simulink model "gm_sampleModel1426_2_sub"  (R2023a)
settings: Solver=VariableStepAuto  StartTime=0.0  StopTime=10.0  RelTol=1e-3
libraries: simulink x2, hdlsllib x1
settings Model: Creator=user1  LastModifiedBy=user1
settings OptimizationCC: BlockReduction=off  ConditionallyExecuteInputs=off
settings DebuggingCC: InheritedTsInSrcMsg=none

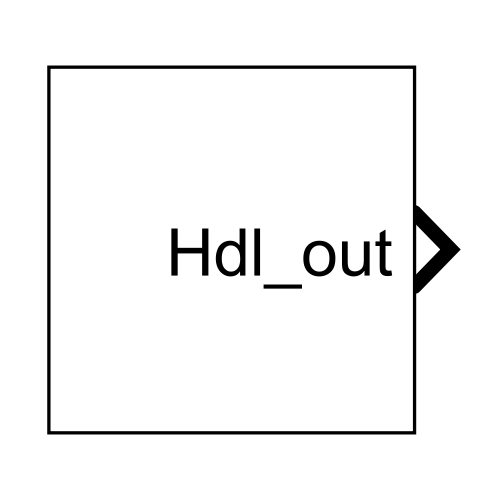
[thumbnail: Simulink's stored preview of the top-level diagram]
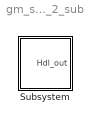
== system gm_sampleModel1426_2_sub ==
  Subsystem : Subsystem

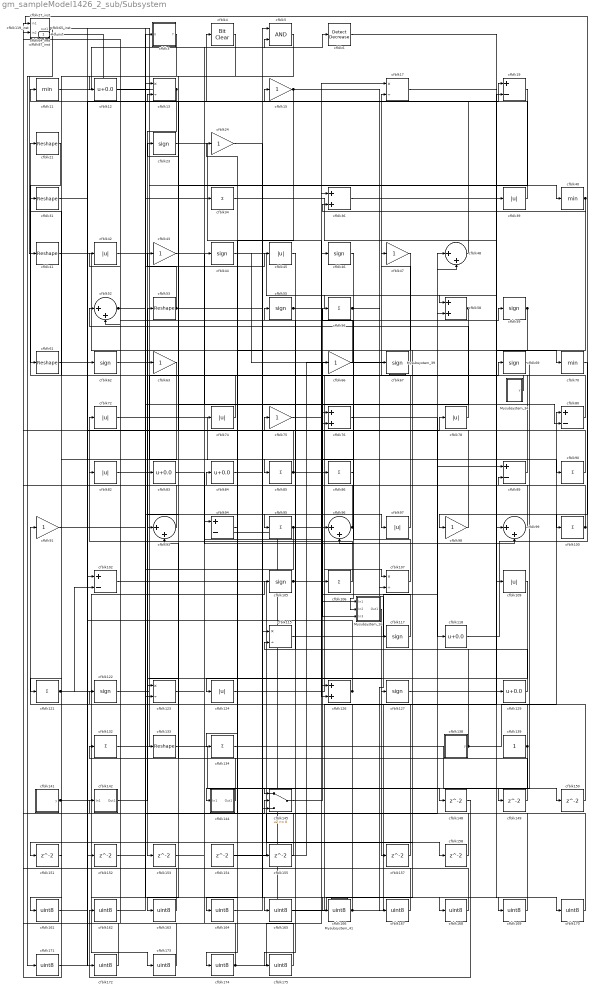
== system gm_sampleModel1426_2_sub/Subsystem ==
  Mysubsystem_16 : Subsystem
  Mysubsystem_34 : Subsystem
  Mysubsystem_39 : Subsystem
  Mysubsystem_41 : Subsystem
  cfblk{34,56,85..86,90,95,100,106,121,132,134} (11 alike) : Sum  Inputs=+  OutDataTypeStr=uint8
  cfblk{19,80,89,94,102} (5 alike) : Sum  Inputs=+-  OutDataTypeStr=uint8
  cfblk{23,44,46,55,59,62,67,69,105,117,122,127} (12 alike) : Signum
  cfblk{13,17,107,115,123} (5 alike) : Product  Inputs=*/  OutDataTypeStr=uint8  RndMeth=Zero  SaturateOnIntegerOverflow=on
  cfblk{39,42,45,72,74,78,82,97,109,124} (10 alike) : Abs  OutDataTypeStr=uint8  SaturateOnIntegerOverflow=off
  cfblk11 : MinMax  OutDataTypeStr=uint8
  cfblk111_inst : Subsystem
  cfblk{12,83..84,118,129} (5 alike) : Bias  Bias=0.0  SaturateOnIntegerOverflow=off
  cfblk119_inst : Subsystem
  cfblk{36,58,76,126} (4 alike) : Sum  OutDataTypeStr=uint8
  cfblk{21,31,41,53,61,133} (6 alike) : Reshape
  cfblk138 : Subsystem  mask(Counter Limited){uplimit=double(7), tsamp=double(-1)}
      mask prompts: uplimit "Simulink:masks:UpperLimit_MP"; tsamp "Simulink:masks:SampleTime_MP"
      mask help: Simulink:masks:CounterLimited_MD
      mask init:
      | nbits = double(8);
      | tsamp = double(-1);
      | uplimit = double(7);
  cfblk139 : Constant  OutDataTypeStr=uint8  SampleTime=-1
  cfblk141 : Subsystem  mask(Counter Free-Running){NumBits=double(16), tsamp=double(-1)}
      mask prompts: NumBits "Simulink:masks:NumberOfBits_MP"; tsamp "Simulink:masks:SampleTime_MP"
      mask help: Simulink:masks:CounterFreeRunning_MD
  cfblk142 : Subsystem
  cfblk144 : Subsystem
  cfblk145 : Switch  OutDataTypeStr=uint8  SaturateOnIntegerOverflow=off  InputSameDT=off
  cfblk{148..155,157..158} (10 alike) : Delay  SampleTime=1
  cfblk{15,24,43,47,63,66,75,91,98} (9 alike) : Gain  OutDataTypeStr=uint8
  cfblk{161..175} (15 alike) : DataTypeConversion  OutDataTypeStr=uint8  SaturateOnIntegerOverflow=off  RndMeth=Floor
  cfblk27_inst : Subsystem
  cfblk3 : Subsystem  mask(Detect Rise Positive){vinit=double(0), InputProcessing=Elements as channels (sample based), OutDataTypeStr=uint8}
      mask prompts: vinit "Simulink:masks:InitialCondition_MP"; InputProcessing "Simulink:masks:InputProcessing_MP"; OutDataTypeStr "Simulink:masks:OutputDataType_MP"
      mask help: Simulink:masks:DetectRisePositive_MD
      mask init:
      | InputProcessing = 'Elements as channels (sample based)';
      | OutDataTypeStr = 'uint8';
      | vinit = double(0);
      mask TypeOptions InputProcessing: Simulink:masks:ColumnsAsChannelsFrameBased | Simulink:masks:ElementsAsChannelsSampleBased
      mask TypeOptions OutDataTypeStr: Simulink:masks:uint8 | Simulink:masks:boolean
      mask Display: fprintf('U > 0\n&  NOT\nU/z > 0')
  cfblk4 : simulink/Logic and Bit Operations/Bit Clear  iBit=0
      settings: LibrarySourceBlock=|
      | hdlsllib/Logic and Bit
      | Operations/Bit Clear
  cfblk40 : MinMax  OutDataTypeStr=uint8
  cfblk{48,52,93,96,99} (5 alike) : Sum  Inputs=|++  OutDataTypeStr=uint8
  cfblk5 : Logic  AllPortsSameDT=off  OutDataTypeStr=boolean
  cfblk6 : simulink/Logic and Bit Operations/Detect Decrease  vinit=0.0  OutDataTypeStr=uint8
      settings: LibrarySourceBlock=|
      | hdlsllib/Logic and Bit
      | Operations/Detect
      | Decrease
  cfblk64_inst : Subsystem
  cfblk65_inst : Subsystem
  cfblk70 : MinMax  OutDataTypeStr=uint8
  cfblk87_inst : Subsystem
  Hdl_out : Outport  OutDataTypeStr=uint8  SampleTime=1
  wires:
  Mysubsystem_16/1(Out1) -> cfblk151/1
  Mysubsystem_34/1(y) -> cfblk21/1
  Mysubsystem_39/1(Out1) -> cfblk154/1
  Mysubsystem_41/1(Out1) -> cfblk94/2
  cfblk100/1 -> cfblk89/2, cfblk98/1
  cfblk102/1 -> cfblk158/1
  cfblk105/1 -> cfblk107/1, Mysubsystem_16/3(In3)
  cfblk106/1 -> cfblk72/1
  cfblk107/1 -> cfblk75/1
  cfblk109/1 -> cfblk124/1
  cfblk11/1 -> cfblk5/2
  cfblk111_inst/1(out1) -> cfblk171/1
  cfblk115/1 -> cfblk48/1
  cfblk117/1 -> cfblk66/1
  cfblk118/1 -> cfblk87_inst/1(in1)
  cfblk119_inst/1(out1) -> cfblk85/1
  cfblk12/1 -> cfblk40/1
  cfblk121/1 -> cfblk105/1, cfblk102/2
  cfblk122/1 -> cfblk127/1
  cfblk123/1 -> cfblk6/1
  cfblk124/1 -> cfblk17/2
  cfblk126/1 -> cfblk46/1, cfblk102/1
  cfblk127/1 -> cfblk39/1
  cfblk129/1 -> cfblk115/2
  cfblk13/1 -> cfblk153/1, Hdl_out/1
  cfblk132/1 -> cfblk67/1
  cfblk133/1 -> cfblk148/1
  cfblk134/1 -> cfblk150/1
  cfblk138/1(y) -> cfblk80/1, cfblk55/1
  cfblk139/1 -> cfblk52/2, cfblk144/1(In1)
  cfblk141/1(y) -> cfblk44/1, cfblk173/1, cfblk168/1, cfblk165/1
  cfblk142/1(Out1) -> cfblk53/1
  cfblk144/1(Out1) -> cfblk132/1
  cfblk145/1 -> cfblk106/1
  cfblk148/1 -> cfblk162/1
  cfblk149/1 -> cfblk93/2
  cfblk15/1 -> cfblk164/1, cfblk107/2
  cfblk150/1 -> cfblk126/1
  cfblk151/1 -> cfblk119_inst/2(in2)
  cfblk152/1 -> cfblk145/2
  cfblk153/1 -> cfblk96/1
  cfblk154/1 -> cfblk48/2
  cfblk155/1 -> cfblk27_inst/1(in1)
  cfblk157/1 -> cfblk115/1
  cfblk158/1 -> cfblk5/1
  cfblk161/1 -> cfblk78/1
  cfblk162/1 -> cfblk3/1(U)
  cfblk163/1 -> cfblk87_inst/2(in2)
  cfblk164/1 -> cfblk19/1
  cfblk165/1 -> cfblk19/2
  cfblk166/1 -> cfblk58/2, cfblk91/1
  cfblk167/1 -> cfblk64_inst/1(in1)
  cfblk168/1 -> cfblk64_inst/2(in2)
  cfblk169/1 -> cfblk142/1(In1)
  cfblk17/1 -> cfblk170/1
  cfblk170/1 -> cfblk84/1
  cfblk171/1 -> cfblk62/1
  cfblk172/1 -> cfblk111_inst/1(in1)
  cfblk173/1 -> cfblk111_inst/2(in2)
  cfblk174/1 -> cfblk76/2, cfblk122/1
  cfblk175/1 -> cfblk94/1
  cfblk19/1 -> cfblk163/1
  cfblk21/1 -> cfblk61/1
  cfblk23/1 -> cfblk126/2
  cfblk24/1 -> cfblk155/1
  cfblk27_inst/1(out1) -> cfblk65_inst/2(in2), cfblk41/1
  cfblk3/1(Y) -> cfblk161/1
  cfblk31/1 -> cfblk172/1
  cfblk34/1 -> cfblk129/1
  cfblk36/1 -> cfblk70/1
  cfblk39/1 -> cfblk4/1
  cfblk4/1 -> cfblk12/1
  cfblk40/1 -> cfblk36/2, Mysubsystem_41/1(In1)
  cfblk41/1 -> cfblk145/3
  cfblk42/1 -> Mysubsystem_39/1(In1)
  cfblk43/1 -> cfblk76/1
  cfblk44/1 -> cfblk109/1
  cfblk45/1 -> cfblk175/1
  cfblk46/1 -> cfblk86/1
  cfblk47/1 -> cfblk145/1
  cfblk48/1 -> cfblk11/1
  cfblk5/1 -> cfblk93/1
  cfblk52/1 -> cfblk83/1, cfblk80/2, cfblk34/1
  cfblk53/1 -> cfblk97/1, cfblk43/1
  cfblk55/1 -> cfblk58/1, Mysubsystem_16/1(In1)
  cfblk56/1 -> cfblk167/1, cfblk117/1
  cfblk58/1 -> cfblk157/1, cfblk123/1
  cfblk59/1 -> Mysubsystem_16/2(In2), cfblk134/1
  cfblk6/1 -> cfblk99/1
  cfblk61/1 -> cfblk15/1
  cfblk62/1 -> cfblk90/1
  cfblk63/1 -> cfblk121/1
  cfblk64_inst/1(out1) -> cfblk166/1
  cfblk65_inst/1(out1) -> cfblk152/1, cfblk95/1
  cfblk66/1 -> cfblk119_inst/1(in1)
  cfblk67/1 -> cfblk47/1
  cfblk69/1 -> cfblk149/1
  cfblk70/1 -> cfblk100/1
  cfblk72/1 -> cfblk118/1
  cfblk74/1 -> cfblk63/1
  cfblk75/1 -> cfblk17/1
  cfblk76/1 -> cfblk89/1
  cfblk78/1 -> cfblk52/1
  cfblk80/1 -> cfblk13/2
  cfblk82/1 -> cfblk133/1
  cfblk83/1 -> cfblk99/2
  cfblk84/1 -> cfblk169/1
  cfblk85/1 -> cfblk69/1, cfblk65_inst/1(in1), cfblk59/1
  cfblk86/1 -> cfblk96/2
  cfblk87_inst/1(out1) -> cfblk74/1
  cfblk89/1 -> cfblk42/1
  cfblk90/1 -> cfblk23/1
  cfblk91/1 -> cfblk45/1
  cfblk93/1 -> cfblk27_inst/2(in2)
  cfblk94/1 -> cfblk174/1
  cfblk95/1 -> cfblk36/1, cfblk123/2
  cfblk96/1 -> cfblk82/1, cfblk56/1
  cfblk97/1 -> cfblk31/1
  cfblk98/1 -> cfblk13/1
  cfblk99/1 -> cfblk24/1

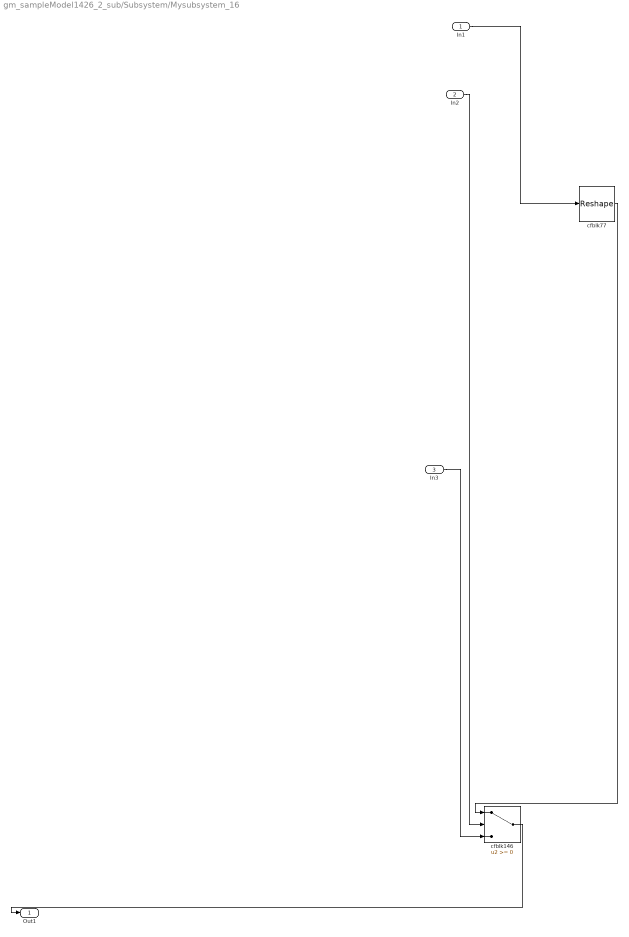
== system gm_sampleModel1426_2_sub/Subsystem/Mysubsystem_16 ==
  In1 : Inport  OutDataTypeStr=uint8  PortDimensions=1  SampleTime=1
  In2 : Inport  Port=2  OutDataTypeStr=uint8  PortDimensions=1  SampleTime=1
  In3 : Inport  Port=3  OutDataTypeStr=uint8  PortDimensions=1  SampleTime=1
  cfblk146 : Switch  SaturateOnIntegerOverflow=off  InputSameDT=off
  cfblk77 : Reshape
  Out1 : Outport  SampleTime=1
  wires:
  In1/1 -> cfblk77/1
  In2/1 -> cfblk146/2
  In3/1 -> cfblk146/3
  cfblk146/1 -> Out1/1
  cfblk77/1 -> cfblk146/1

== system gm_sampleModel1426_2_sub/Subsystem/Mysubsystem_34 ==
  cfblk140 : Subsystem  mask(Counter Free-Running){NumBits=double(16), tsamp=double(-1)}
      mask prompts: NumBits "Simulink:masks:NumberOfBits_MP"; tsamp "Simulink:masks:SampleTime_MP"
      mask help: Simulink:masks:CounterFreeRunning_MD
  cfblk8 : hdlsllib/Logic and Bit Operations/Interval Test  IntervalClosedRight=on  uplimit=0.5  IntervalClosedLeft=on  lowlimit=-0.5  OutDataTypeStr=boolean
  y : Outport  SampleTime=1
  wires:
  cfblk140/1(y) -> cfblk8/1
  cfblk8/1 -> y/1

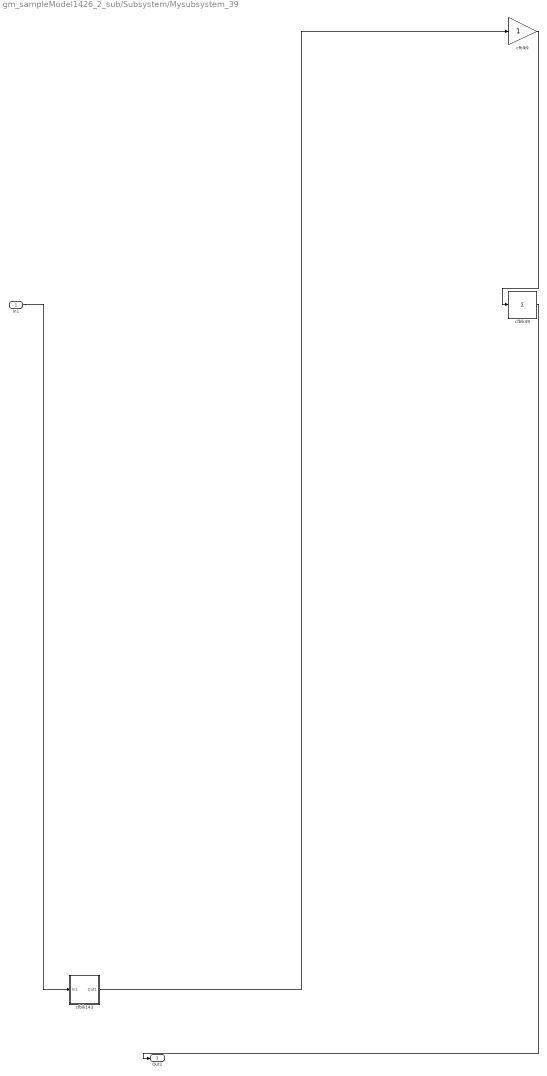
== system gm_sampleModel1426_2_sub/Subsystem/Mysubsystem_39 ==
  In1 : Inport  OutDataTypeStr=uint8  PortDimensions=1  SampleTime=1
  cfblk143 : Subsystem
  cfblk49 : Sum  Inputs=+
  cfblk9 : Gain
  Out1 : Outport  SampleTime=1
  wires:
  In1/1 -> cfblk143/1(In1)
  cfblk143/1(Out1) -> cfblk9/1
  cfblk49/1 -> Out1/1
  cfblk9/1 -> cfblk49/1

== system gm_sampleModel1426_2_sub/Subsystem/Mysubsystem_41 ==
  In1 : Inport  OutDataTypeStr=uint8  PortDimensions=1  SampleTime=1
  cfblk156 : Delay  SampleTime=1
  cfblk176 : DataTypeConversion  OutDataTypeStr=uint8  SaturateOnIntegerOverflow=off  RndMeth=Floor
  Out1 : Outport  SampleTime=1
  wires:
  In1/1 -> cfblk156/1
  cfblk156/1 -> cfblk176/1
  cfblk176/1 -> Out1/1

== system gm_sampleModel1426_2_sub/Subsystem/cfblk111_inst ==
  in1 : Inport  OutDataTypeStr=uint8  SampleTime=1
  in2 : Inport  Port=2  OutDataTypeStr=uint8  SampleTime=1
  mul_cfblk111_dotp_mulcomp : Product  Inputs=**  OutDataTypeStr=uint8  SampleTime=1
  out1 : Outport  OutDataTypeStr=uint8  SampleTime=1
  wires:
  in1/1 -> mul_cfblk111_dotp_mulcomp/1
  in2/1 -> mul_cfblk111_dotp_mulcomp/2
  mul_cfblk111_dotp_mulcomp/1 -> out1/1

== system gm_sampleModel1426_2_sub/Subsystem/cfblk119_inst ==
  in1 : Inport  OutDataTypeStr=uint8  SampleTime=1
  in2 : Inport  Port=2  OutDataTypeStr=uint8  SampleTime=1
  mul_cfblk119_dotp_mulcomp : Product  Inputs=**  OutDataTypeStr=uint8  SampleTime=1
  out1 : Outport  OutDataTypeStr=uint8  SampleTime=1
  wires:
  in1/1 -> mul_cfblk119_dotp_mulcomp/1
  in2/1 -> mul_cfblk119_dotp_mulcomp/2
  mul_cfblk119_dotp_mulcomp/1 -> out1/1

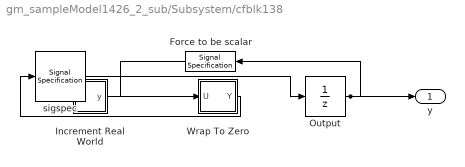
== system gm_sampleModel1426_2_sub/Subsystem/cfblk138 ==
  Force to be scalar : SignalSpecification  DisableCoverage=on  Dimensions=1
  Increment Real World : Subsystem  mask(Real World Value Increment){}
      mask help: Simulink:masks:RealWorldValueIncrement_MD
      mask Display: disp('V++')
  Output : UnitDelay  InitialCondition=0.0  SampleTime=tsamp  HasFrameUpgradeWarning=on
  Wrap To Zero : Subsystem  mask(Wrap To Zero){Threshold=double(7)}
      mask prompts: Threshold "Simulink:masks:Threshold_MP"
      mask help: Simulink:masks:WrapToZero_MD
  sigspec : SignalSpecification  OutDataTypeStr=uint8  Dimensions=1
  y : Outport  SampleTime=1
  wires:
  Force to be scalar/1 -> Increment Real World/1(u)
  Increment Real World/1(y) -> Wrap To Zero/1(U)
  Output/1 -> Force to be scalar/1, y/1
  Wrap To Zero/1(Y) -> sigspec/1
  sigspec/1 -> Output/1

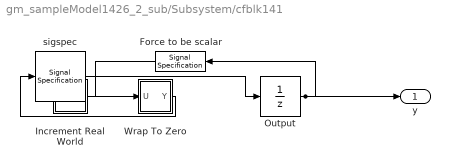
== system gm_sampleModel1426_2_sub/Subsystem/cfblk141 ==
  Force to be scalar : SignalSpecification  DisableCoverage=on  Dimensions=1
  Increment Real World : Subsystem  mask(Real World Value Increment){}
      mask help: Simulink:masks:RealWorldValueIncrement_MD
      mask Display: disp('V++')
  Output : UnitDelay  InitialCondition=0.0  SampleTime=tsamp  HasFrameUpgradeWarning=on
  Wrap To Zero : Subsystem  mask(Wrap To Zero){Threshold=double(65535)}
      mask prompts: Threshold "Simulink:masks:Threshold_MP"
      mask help: Simulink:masks:WrapToZero_MD
  sigspec : SignalSpecification  OutDataTypeStr=uint16  Dimensions=1
  y : Outport  SampleTime=1
  wires:
  Force to be scalar/1 -> Increment Real World/1(u)
  Increment Real World/1(y) -> Wrap To Zero/1(U)
  Output/1 -> Force to be scalar/1, y/1
  Wrap To Zero/1(Y) -> sigspec/1
  sigspec/1 -> Output/1

== system gm_sampleModel1426_2_sub/Subsystem/cfblk142 ==
  In1 : Inport  OutDataTypeStr=uint8  PortDimensions=1  SampleTime=1
  Out1 : Outport  SampleTime=1
  wires:
  In1/1 -> Out1/1

== system gm_sampleModel1426_2_sub/Subsystem/cfblk144 ==
  In1 : Inport  OutDataTypeStr=uint8  PortDimensions=1  SampleTime=1
  Out1 : Outport  SampleTime=1
  wires:
  In1/1 -> Out1/1

== system gm_sampleModel1426_2_sub/Subsystem/cfblk27_inst ==
  in1 : Inport  OutDataTypeStr=uint8  SampleTime=1
  in2 : Inport  Port=2  OutDataTypeStr=uint8  SampleTime=1
  mul_cfblk27_dotp_mulcomp : Product  Inputs=**  OutDataTypeStr=uint8  SampleTime=1
  out1 : Outport  OutDataTypeStr=uint8  SampleTime=1
  wires:
  in1/1 -> mul_cfblk27_dotp_mulcomp/1
  in2/1 -> mul_cfblk27_dotp_mulcomp/2
  mul_cfblk27_dotp_mulcomp/1 -> out1/1

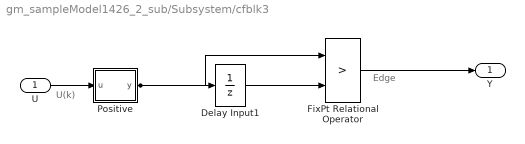
== system gm_sampleModel1426_2_sub/Subsystem/cfblk3 ==
  note: U(k)
  note: Edge
  U : Inport  OutDataTypeStr=uint8  SampleTime=1
  Delay Input1 : UnitDelay  Description=Store in Global RAM  DisableCoverage=on  InitialCondition=vinit  SampleTime=-1  HasFrameUpgradeWarning=on
  FixPt Relational Operator : RelationalOperator  Operator=>  OutDataTypeStr=fixdt(0, 8)  ZeroCross=off  InputSameDT=off
  Positive : Subsystem  mask(Compare To Zero){relop=>, OutDataTypeStr=boolean, ZeroCross=off}
      mask prompts: relop "Simulink:masks:Operator_MP"; OutDataTypeStr "Simulink:masks:OutputDataType_MP"; ZeroCross "Simulink:masks:EnableZerocrossingDetection_MP"
      mask help: Simulink:masks:CompareToZero_MD
      mask init:
      | OutDataTypeStr = 'boolean';
      | ZeroCross = 'off';
      | blkName = 'sampleModel1426_2_sub/Subsystem/cfblk3/Positive';
      | relop = '>';
      | setValue = 'boolean';
      mask TypeOptions relop: == | ~= | < | <= | >= | >
      mask TypeOptions OutDataTypeStr: Simulink:masks:uint8 | Simulink:masks:boolean
      mask Callback ZeroCross: sl('zeroCrossEnable', gcbh);
      mask Display: disp([relop,' 0'])
  Y : Outport  SampleTime=1
  wires:
  U/1 -> Positive/1(u)
  Delay Input1/1 -> FixPt Relational Operator/2
  FixPt Relational Operator/1 -> Y/1
  Positive/1(y) -> FixPt Relational Operator/1, Delay Input1/1

== system gm_sampleModel1426_2_sub/Subsystem/cfblk64_inst ==
  in1 : Inport  OutDataTypeStr=uint8  SampleTime=1
  in2 : Inport  Port=2  OutDataTypeStr=uint8  SampleTime=1
  mul_cfblk64_dotp_mulcomp : Product  Inputs=**  OutDataTypeStr=uint8  SampleTime=1
  out1 : Outport  OutDataTypeStr=uint8  SampleTime=1
  wires:
  in1/1 -> mul_cfblk64_dotp_mulcomp/1
  in2/1 -> mul_cfblk64_dotp_mulcomp/2
  mul_cfblk64_dotp_mulcomp/1 -> out1/1

== system gm_sampleModel1426_2_sub/Subsystem/cfblk65_inst ==
  in1 : Inport  OutDataTypeStr=uint8  SampleTime=1
  in2 : Inport  Port=2  OutDataTypeStr=uint8  SampleTime=1
  mul_cfblk65_dotp_mulcomp : Product  Inputs=**  OutDataTypeStr=uint8  SampleTime=1
  out1 : Outport  OutDataTypeStr=uint8  SampleTime=1
  wires:
  in1/1 -> mul_cfblk65_dotp_mulcomp/1
  in2/1 -> mul_cfblk65_dotp_mulcomp/2
  mul_cfblk65_dotp_mulcomp/1 -> out1/1

== system gm_sampleModel1426_2_sub/Subsystem/cfblk87_inst ==
  in1 : Inport  OutDataTypeStr=uint8  SampleTime=1
  in2 : Inport  Port=2  OutDataTypeStr=uint8  SampleTime=1
  mul_cfblk87_dotp_mulcomp : Product  Inputs=**  OutDataTypeStr=uint8  SampleTime=1
  out1 : Outport  OutDataTypeStr=uint8  SampleTime=1
  wires:
  in1/1 -> mul_cfblk87_dotp_mulcomp/1
  in2/1 -> mul_cfblk87_dotp_mulcomp/2
  mul_cfblk87_dotp_mulcomp/1 -> out1/1

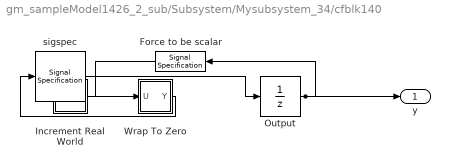
== system gm_sampleModel1426_2_sub/Subsystem/Mysubsystem_34/cfblk140 ==
  Force to be scalar : SignalSpecification  DisableCoverage=on  Dimensions=1
  Increment Real World : Subsystem  mask(Real World Value Increment){}
      mask help: Simulink:masks:RealWorldValueIncrement_MD
      mask Display: disp('V++')
  Output : UnitDelay  InitialCondition=0.0  SampleTime=tsamp  HasFrameUpgradeWarning=on
  Wrap To Zero : Subsystem  mask(Wrap To Zero){Threshold=double(65535)}
      mask prompts: Threshold "Simulink:masks:Threshold_MP"
      mask help: Simulink:masks:WrapToZero_MD
  sigspec : SignalSpecification  OutDataTypeStr=uint16  Dimensions=1
  y : Outport  SampleTime=1
  wires:
  Force to be scalar/1 -> Increment Real World/1(u)
  Increment Real World/1(y) -> Wrap To Zero/1(U)
  Output/1 -> Force to be scalar/1, y/1
  Wrap To Zero/1(Y) -> sigspec/1
  sigspec/1 -> Output/1

== system gm_sampleModel1426_2_sub/Subsystem/Mysubsystem_39/cfblk143 ==
  In1 : Inport  OutDataTypeStr=uint8  PortDimensions=1  SampleTime=1
  Out1 : Outport  SampleTime=1
  wires:
  In1/1 -> Out1/1

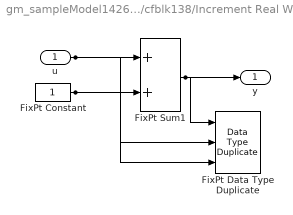
== system gm_sampleModel1426_2_sub/Subsystem/cfblk138/Increment Real World ==
  u : Inport  OutDataTypeStr=uint8  SampleTime=1
  FixPt Constant : Constant  DisableCoverage=on  OutDataTypeStr=Inherit: Inherit via back propagation  SampleTime=-1
  FixPt Data Type Duplicate : DataTypeDuplicate  DisableCoverage=on  NumInputPorts=3
  FixPt Sum1 : Sum  InputSameDT=on  OutDataTypeStr=Inherit: Inherit via back propagation  LockScale=on
  y : Outport  SampleTime=1
  wires:
  u/1 -> FixPt Sum1/1, FixPt Data Type Duplicate/2
  FixPt Constant/1 -> FixPt Sum1/2, FixPt Data Type Duplicate/3
  FixPt Sum1/1 -> FixPt Data Type Duplicate/1, y/1

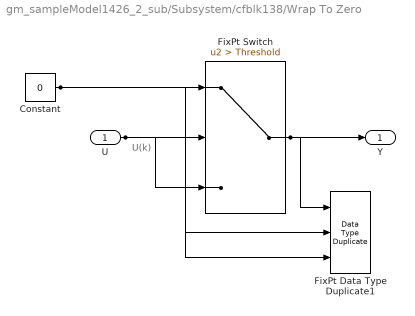
== system gm_sampleModel1426_2_sub/Subsystem/cfblk138/Wrap To Zero ==
  note: U(k)
  U : Inport  OutDataTypeStr=uint8  SampleTime=1
  Constant : Constant  DisableCoverage=on  Value=0  OutDataTypeStr=Inherit: Inherit via back propagation  SampleTime=-1
  FixPt Data Type Duplicate1 : DataTypeDuplicate  DisableCoverage=on  NumInputPorts=3
  FixPt Switch : Switch  Criteria=u2 > Threshold  Threshold=Threshold  OutDataTypeStr=Inherit: Inherit via back propagation  ZeroCross=off  SaturateOnIntegerOverflow=off  InputSameDT=off
  Y : Outport  SampleTime=1
  wires:
  U/1 -> FixPt Switch/3, FixPt Switch/2, FixPt Data Type Duplicate1/2
  Constant/1 -> FixPt Switch/1, FixPt Data Type Duplicate1/3
  FixPt Switch/1 -> FixPt Data Type Duplicate1/1, Y/1

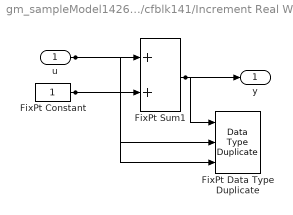
== system gm_sampleModel1426_2_sub/Subsystem/cfblk141/Increment Real World ==
  u : Inport  OutDataTypeStr=uint16  SampleTime=1
  FixPt Constant : Constant  DisableCoverage=on  OutDataTypeStr=Inherit: Inherit via back propagation  SampleTime=-1
  FixPt Data Type Duplicate : DataTypeDuplicate  DisableCoverage=on  NumInputPorts=3
  FixPt Sum1 : Sum  InputSameDT=on  OutDataTypeStr=Inherit: Inherit via back propagation  LockScale=on
  y : Outport  SampleTime=1
  wires:
  u/1 -> FixPt Sum1/1, FixPt Data Type Duplicate/2
  FixPt Constant/1 -> FixPt Sum1/2, FixPt Data Type Duplicate/3
  FixPt Sum1/1 -> FixPt Data Type Duplicate/1, y/1

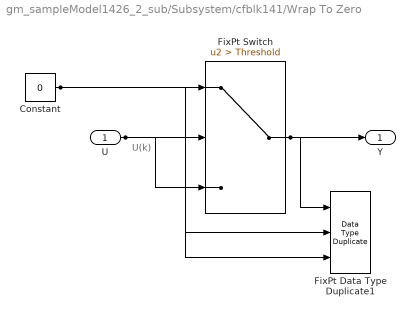
== system gm_sampleModel1426_2_sub/Subsystem/cfblk141/Wrap To Zero ==
  note: U(k)
  U : Inport  OutDataTypeStr=uint16  SampleTime=1
  Constant : Constant  DisableCoverage=on  Value=0  OutDataTypeStr=Inherit: Inherit via back propagation  SampleTime=-1
  FixPt Data Type Duplicate1 : DataTypeDuplicate  DisableCoverage=on  NumInputPorts=3
  FixPt Switch : Switch  Criteria=u2 > Threshold  Threshold=Threshold  OutDataTypeStr=Inherit: Inherit via back propagation  ZeroCross=off  SaturateOnIntegerOverflow=off  InputSameDT=off
  Y : Outport  SampleTime=1
  wires:
  U/1 -> FixPt Switch/3, FixPt Switch/2, FixPt Data Type Duplicate1/2
  Constant/1 -> FixPt Switch/1, FixPt Data Type Duplicate1/3
  FixPt Switch/1 -> FixPt Data Type Duplicate1/1, Y/1

== system gm_sampleModel1426_2_sub/Subsystem/cfblk3/Positive ==
  u : Inport  OutDataTypeStr=uint8  SampleTime=1
  Compare : RelationalOperator  Operator=>  OutDataTypeStr=boolean  ZeroCross=off
  Constant : Constant  DisableCoverage=on  Value=0  OutDataTypeStr=Inherit: Inherit via back propagation  SampleTime=-1  PreserveConstantTs=on
  y : Outport  SampleTime=1
  wires:
  u/1 -> Compare/1
  Compare/1 -> y/1
  Constant/1 -> Compare/2

== system gm_sampleModel1426_2_sub/Subsystem/Mysubsystem_34/cfblk140/Increment Real World ==
  u : Inport  OutDataTypeStr=uint16  SampleTime=1
  FixPt Constant : Constant  DisableCoverage=on  OutDataTypeStr=Inherit: Inherit via back propagation  SampleTime=-1
  FixPt Data Type Duplicate : DataTypeDuplicate  DisableCoverage=on  NumInputPorts=3
  FixPt Sum1 : Sum  InputSameDT=on  OutDataTypeStr=Inherit: Inherit via back propagation  LockScale=on
  y : Outport  SampleTime=1
  wires:
  u/1 -> FixPt Sum1/1, FixPt Data Type Duplicate/2
  FixPt Constant/1 -> FixPt Sum1/2, FixPt Data Type Duplicate/3
  FixPt Sum1/1 -> FixPt Data Type Duplicate/1, y/1

== system gm_sampleModel1426_2_sub/Subsystem/Mysubsystem_34/cfblk140/Wrap To Zero ==
  note: U(k)
  U : Inport  OutDataTypeStr=uint16  SampleTime=1
  Constant : Constant  DisableCoverage=on  Value=0  OutDataTypeStr=Inherit: Inherit via back propagation  SampleTime=-1
  FixPt Data Type Duplicate1 : DataTypeDuplicate  DisableCoverage=on  NumInputPorts=3
  FixPt Switch : Switch  Criteria=u2 > Threshold  Threshold=Threshold  OutDataTypeStr=Inherit: Inherit via back propagation  ZeroCross=off  SaturateOnIntegerOverflow=off  InputSameDT=off
  Y : Outport  SampleTime=1
  wires:
  U/1 -> FixPt Switch/3, FixPt Switch/2, FixPt Data Type Duplicate1/2
  Constant/1 -> FixPt Switch/1, FixPt Data Type Duplicate1/3
  FixPt Switch/1 -> FixPt Data Type Duplicate1/1, Y/1
